simulink model "line_following_2023a"  (R2023a)
settings: Solver=ode1  StartTime=0.0  StopTime=inf  FixedStep=1/60  RelTol=1e-3  EnableMultiTasking=on
model workspace (MAT data in the model file):
  downCamStepSize : Simulink.Parameter (value not decoded)
  lidarStepSize : Simulink.Parameter (value not decoded)
  mainStepSize : Simulink.Parameter (value not decoded)
  mode : Simulink.Parameter (value not decoded)
  realSenseStepSize : Simulink.Parameter (value not decoded)
symbols that are objects in the model workspace (value not decoded): downCamStepSize, mainStepSize, mode
undefined symbols (not defined in the file or in its folder): gcbh, JPEG, video_display_show
libraries: quarc_library x53
(part 2 of 2)

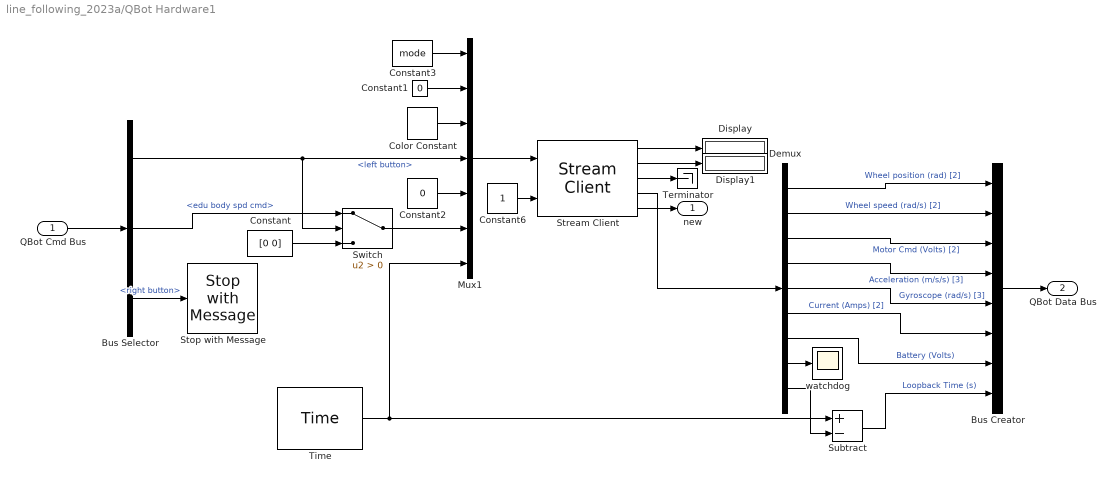
== system line_following_2023a/QBot Hardware1 ==
  QBot Cmd Bus : Inport
  Bus Creator : BusCreator  Inputs=8
  Bus Selector : BusSelector  OutputSignals=left button,edu body spd cmd,right button
  Color Constant : quarc_library/Sources/Signals/Color Constant  color=[0 1 1]
      settings: SourceProductName=QUARC Targets
  Constant : Constant  Value=[0 0]
  Constant1 : Constant  Value=0
  Constant2 : Constant  Value=0
  Constant3 : Constant  Value=mode
  Constant6 : Constant
  Demux : Demux  Outputs=[2 2 2 3 3 2 1 1 1]
  Display : Display
  Display1 : Display
  Mux1 : Mux  Inputs=7
  Stop with Message : quarc_library/Sinks/Error Handling/Stop with Message  message_type=Fixed error message  message_icon=Information  message=Operator: Emergency Stop
  Stream Client : quarc_library/Communications/Basic/Stream Client  uri_source=Specify via dialog (do not evaluate)  uri=tcpip://localhost:18971  send_buffer_size=1460  receive_buffer_size=1460  byte_order=little endian (Intel - LSB first)  optimization=Minimum latency  send_options=Send most recent data  receive_options=Receive most recent data  default_value=zeros(17,1)  sample_time=qc_get_step_size  active=on  implementation=Use blocking I/O in a separate thread  send_fifo_size=1000  receive_fifo_size=1000  send_priority=0  receive_priority=0  send_dimensions=off  receive_dimensions=off  max_dimensions=-1  data_type=Inherited via back propagation  type_expr=BusObject
      settings: AttributesFormatString="\"tcpip://localhost:18971\""
  Subtract : Sum  Inputs=+-
  Switch : Switch  Criteria=u2 > Threshold  SaturateOnIntegerOverflow=off  InputSameDT=off
  Terminator : Terminator
  Time : quarc_library/Sources/Time/Time  time_source=Wall clock  sample_time=qc_get_step_size
  watchdog : Scope
  new : Outport
  QBot Data Bus : Outport  Port=2
  wires:
  Demux/2 -> Bus Creator/2  "Wheel speed (rad/s) [2]"
  Constant3/1 -> Mux1/1
  Stream Client/3 -> Terminator/1
  Bus Selector/2 -> Switch/1  "<edu body spd cmd>"
  Stream Client/1 -> Display/1
  Constant6/1 -> Stream Client/2
  Stream Client/2 -> Display1/1
  Color Constant/1 -> Mux1/3
  Constant1/1 -> Mux1/2
  Demux/3 -> Bus Creator/3  "Motor Cmd (Volts) [2]"
  Mux1/1 -> Stream Client/1
  Stream Client/4 -> Demux/1
  Demux/1 -> Bus Creator/1  "Wheel position (rad) [2]"
  Stream Client/5 -> new/1
  Demux/7 -> Bus Creator/7  "Battery (Volts)"
  Demux/5 -> Bus Creator/5  "Gyroscope (rad/s) [3]"
  Demux/6 -> Bus Creator/6  "Current (Amps) [2]"
  Demux/9 -> Subtract/2
  Constant2/1 -> Mux1/5
  Demux/4 -> Bus Creator/4  "Acceleration (m/s/s) [3]"
  Time/1 -> Mux1/7, Subtract/1
  Bus Creator/1 -> QBot Data Bus/1
  Subtract/1 -> Bus Creator/8  "Loopback Time (s)"
  Demux/8 -> watchdog/1
  Switch/1 -> Mux1/6
  Constant/1 -> Switch/3
  QBot Cmd Bus/1 -> Bus Selector/1
  Bus Selector/1 -> Switch/2, Mux1/4  "<left button>"
  Bus Selector/3 -> Stop with Message/1  "<right button>"

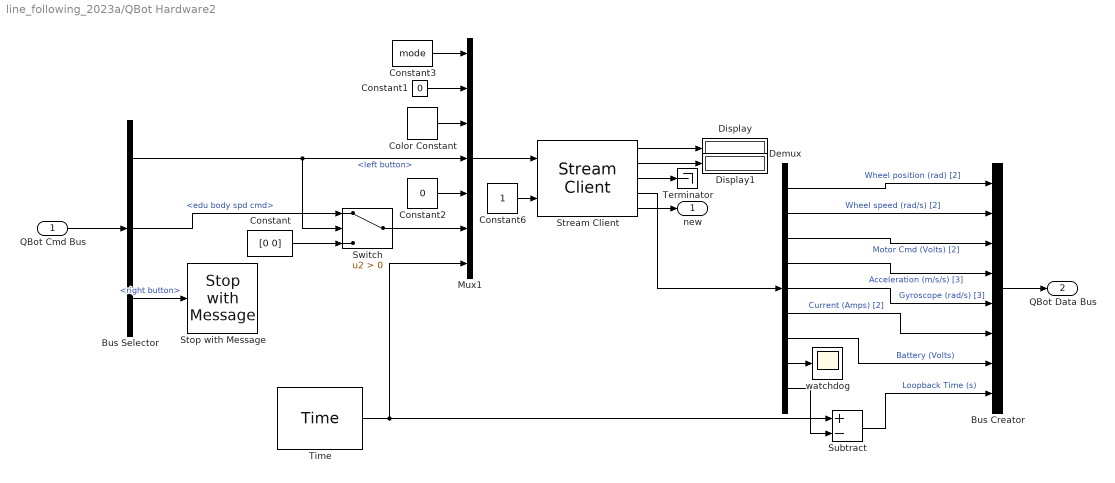
== system line_following_2023a/QBot Hardware2 ==
  QBot Cmd Bus : Inport
  Bus Creator : BusCreator  Inputs=8
  Bus Selector : BusSelector  OutputSignals=left button,edu body spd cmd,right button
  Color Constant : quarc_library/Sources/Signals/Color Constant  color=[0 1 1]
      settings: SourceProductName=QUARC Targets
  Constant : Constant  Value=[0 0]
  Constant1 : Constant  Value=0
  Constant2 : Constant  Value=0
  Constant3 : Constant  Value=mode
  Constant6 : Constant
  Demux : Demux  Outputs=[2 2 2 3 3 2 1 1 1]
  Display : Display
  Display1 : Display
  Mux1 : Mux  Inputs=7
  Stop with Message : quarc_library/Sinks/Error Handling/Stop with Message  message_type=Fixed error message  message_icon=Information  message=Operator: Emergency Stop
  Stream Client : quarc_library/Communications/Basic/Stream Client  uri_source=Specify via dialog (do not evaluate)  uri=tcpip://localhost:18972  send_buffer_size=1460  receive_buffer_size=1460  byte_order=little endian (Intel - LSB first)  optimization=Minimum latency  send_options=Send most recent data  receive_options=Receive most recent data  default_value=zeros(17,1)  sample_time=qc_get_step_size  active=on  implementation=Use blocking I/O in a separate thread  send_fifo_size=1000  receive_fifo_size=1000  send_priority=0  receive_priority=0  send_dimensions=off  receive_dimensions=off  max_dimensions=-1  data_type=Inherited via back propagation  type_expr=BusObject
      settings: AttributesFormatString="\"tcpip://localhost:18972\""
  Subtract : Sum  Inputs=+-
  Switch : Switch  Criteria=u2 > Threshold  SaturateOnIntegerOverflow=off  InputSameDT=off
  Terminator : Terminator
  Time : quarc_library/Sources/Time/Time  time_source=Wall clock  sample_time=qc_get_step_size
  watchdog : Scope
  new : Outport
  QBot Data Bus : Outport  Port=2
  wires:
  Demux/2 -> Bus Creator/2  "Wheel speed (rad/s) [2]"
  Constant3/1 -> Mux1/1
  Stream Client/3 -> Terminator/1
  Bus Selector/2 -> Switch/1  "<edu body spd cmd>"
  Stream Client/1 -> Display/1
  Constant6/1 -> Stream Client/2
  Stream Client/2 -> Display1/1
  Color Constant/1 -> Mux1/3
  Constant1/1 -> Mux1/2
  Demux/3 -> Bus Creator/3  "Motor Cmd (Volts) [2]"
  Mux1/1 -> Stream Client/1
  Stream Client/4 -> Demux/1
  Demux/1 -> Bus Creator/1  "Wheel position (rad) [2]"
  Stream Client/5 -> new/1
  Demux/7 -> Bus Creator/7  "Battery (Volts)"
  Demux/5 -> Bus Creator/5  "Gyroscope (rad/s) [3]"
  Demux/6 -> Bus Creator/6  "Current (Amps) [2]"
  Demux/9 -> Subtract/2
  Constant2/1 -> Mux1/5
  Demux/4 -> Bus Creator/4  "Acceleration (m/s/s) [3]"
  Time/1 -> Mux1/7, Subtract/1
  Bus Creator/1 -> QBot Data Bus/1
  Subtract/1 -> Bus Creator/8  "Loopback Time (s)"
  Demux/8 -> watchdog/1
  Switch/1 -> Mux1/6
  Constant/1 -> Switch/3
  QBot Cmd Bus/1 -> Bus Selector/1
  Bus Selector/1 -> Switch/2, Mux1/4  "<left button>"
  Bus Selector/3 -> Stop with Message/1  "<right button>"

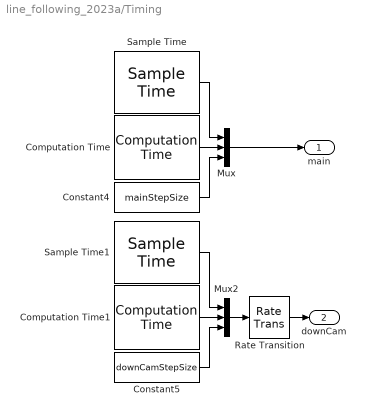
== system line_following_2023a/Timing ==
  Computation Time : quarc_library/Sources/Time/Computation Time  sample_time=mainStepSize  use_model=on  use_cpu_time=off
  Computation Time1 : quarc_library/Sources/Time/Computation Time  sample_time=downCamStepSize  use_model=on  use_cpu_time=off
  Constant4 : Constant  Value=mainStepSize
  Constant5 : Constant  Value=downCamStepSize
  Mux : Mux  Inputs=3
  Mux2 : Mux  Inputs=3
  Rate Transition : RateTransition
  Sample Time : quarc_library/Sources/Time/Sample Time  Priority=-99  sample_time=mainStepSize
  Sample Time1 : quarc_library/Sources/Time/Sample Time  Priority=-99  sample_time=downCamStepSize
  main : Outport
  downCam : Outport  Port=2
  wires:
  Constant5/1 -> Mux2/3
  Computation Time/1 -> Mux/2
  Sample Time/1 -> Mux/1
  Sample Time1/1 -> Mux2/1
  Computation Time1/1 -> Mux2/2
  Constant4/1 -> Mux/3
  Mux2/1 -> Rate Transition/1
  Rate Transition/1 -> downCam/1
  Mux/1 -> main/1

== system line_following_2023a/Image Processing3/Video Compressed Display3 ==
  In1 : Inport
  Channel : quarc_library/Signal Routing/Channel  channel=4  buffer_size=1
  Image Compress : quarc_library/Image Processing/Generic/Image Compress  algorithm=JPEG  source=Internal dialog parameter  quality=quality  output_dim=-1
  Video Display : quarc_library/Multimedia/Video Display  Tag=line_following_2023a/Image Processing3/Video Compressed Display3/Video Display  sample_time=sample_time  use_hardware=on
  wires:
  Channel/1 -> Video Display/1
  In1/1 -> Image Compress/1
  Image Compress/1 -> Channel/1

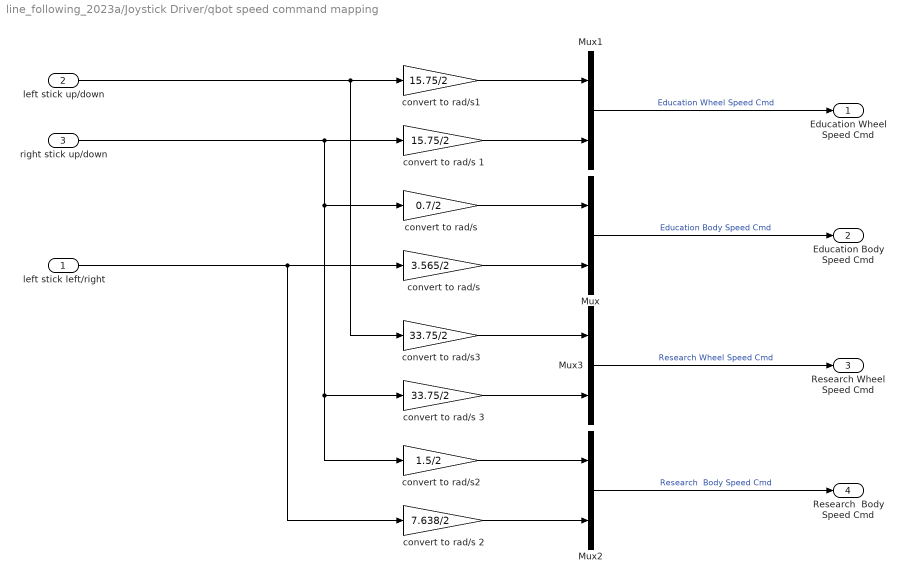
== system line_following_2023a/Joystick Driver/qbot speed command mapping ==
  left stick left/right : Inport
  left stick up/down : Inport  Port=2
  right stick up/down : Inport  Port=3
  Mux{,1..3} (4 alike) : Mux  Inputs=2
  convert to rad/s : Gain  Gain=0.7/2
  "convert to rad/s " : Gain  Gain=3.565/2
  convert to rad/s 1 : Gain  Gain=15.75/2
  convert to rad/s 2 : Gain  Gain=7.638/2
  convert to rad/s 3 : Gain  Gain=33.75/2
  convert to rad/s1 : Gain  Gain=15.75/2
  convert to rad/s2 : Gain  Gain=1.5/2
  convert to rad/s3 : Gain  Gain=33.75/2
  Education Wheel Speed Cmd : Outport
  Education Body Speed Cmd : Outport  Port=2
  Research Wheel Speed Cmd : Outport  Port=3
  Research  Body Speed Cmd : Outport  Port=4
  wires:
  convert to rad/s/1 -> Mux/1
  Mux/1 -> Education Body Speed Cmd/1  "Education Body Speed Cmd"
  left stick left/right/1 -> convert to rad/s 2/1, "convert to rad/s "/1
  convert to rad/s2/1 -> Mux2/1
  left stick up/down/1 -> convert to rad/s3/1, convert to rad/s1/1
  right stick up/down/1 -> convert to rad/s 3/1, convert to rad/s2/1, convert to rad/s/1, convert to rad/s 1/1
  "convert to rad/s "/1 -> Mux/2
  convert to rad/s 3/1 -> Mux3/2
  convert to rad/s3/1 -> Mux3/1
  convert to rad/s 2/1 -> Mux2/2
  convert to rad/s 1/1 -> Mux1/2
  convert to rad/s1/1 -> Mux1/1
  Mux3/1 -> Research Wheel Speed Cmd/1  "Research Wheel Speed Cmd"
  Mux1/1 -> Education Wheel Speed Cmd/1  "Education Wheel Speed Cmd"
  Mux2/1 -> Research  Body Speed Cmd/1  "Research  Body Speed Cmd"

== matlab function line_following_2023a/Joystick Driver/MATLAB Function ==
  data: u input; N output; S output; E output; W output
function [N, S, E, W] = fcn(u)

N = 0;
S = 0;
E = 0;
W = 0;

switch u
    case 0
        N = 1;
    case 3.142
        S = 1;
    case 4.712
        W = 1;
    case 1.571
        E = 1;
    case 3.927
        S = 1;
        W = 1;
    case 2.356
        S = 1;
        E = 1;
    case 0.7854
        N = 1;
        E = 1;
    case 5.498
        N = 1;
        W = 1;
end

== matlab function line_following_2023a/Image Processing1/colorize ==
  data: Binary input; y output; Color input
function y = fcn(Binary, Color)

y = Color;
[ROW, COL, ~] = size(y);

y(51:100, 1:COL, 1) = ((255 - Binary)/255).*Color(51:100,:,1) + (Binary).*Color(51:100, :, 1);
y(51:100, 1:COL, 2) = ((255 - Binary)/255).*Color(51:100,:,2);
y(51:100, 1:COL, 3) = ((255 - Binary)/255).*Color(51:100,:,3);

== matlab function line_following_2023a/Image Processing3/colorize ==
  data: Binary input; y output; Color input
function y = fcn(Binary, Color)

y = Color;
[ROW, COL, ~] = size(y);

y(51:100, 1:COL, 1) = ((255 - Binary)/255).*Color(51:100,:,1) + (Binary).*Color(51:100, :, 1);
y(51:100, 1:COL, 2) = ((255 - Binary)/255).*Color(51:100,:,2);
y(51:100, 1:COL, 3) = ((255 - Binary)/255).*Color(51:100,:,3);

== matlab function line_following_2023a/Image Processing/colorize ==
  data: Binary input; y output; Color input
function y = fcn(Binary, Color)

y = Color;
[ROW, COL, ~] = size(y);

y(51:100, 1:COL, 1) = ((255 - Binary)/255).*Color(51:100,:,1) + (Binary).*Color(51:100, :, 1);
y(51:100, 1:COL, 2) = ((255 - Binary)/255).*Color(51:100,:,2);
y(51:100, 1:COL, 3) = ((255 - Binary)/255).*Color(51:100,:,3);
